simulink model "flightController"  (R2021b)
settings: Solver=ode3  StartTime=0  StopTime=10.0  FixedStep=Ts  RelTol=1e-3  EnableMultiTasking=on
settings Model: Creator=The MathWorks, Inc.  LastModifiedBy=Tiga
settings SolverCC: AlgebraicLoopSolver=TrustRegion  AutoInsertRateTranBlk=on
settings DataIOCC: SaveFormat=Array  ReturnWorkspaceOutputs=off
settings OptimizationCC: BlockReduction=off  DefaultParameterBehavior=Inlined  BufferReuse=off  LifeSpan=inf
settings DebuggingCC: AlgebraicLoopMsg=none  UnderspecifiedInitializationDetection=Classic  MergeDetectMultiDrivingBlocksExec=none  UnconnectedInputMsg=none  UnconnectedOutputMsg=none  UnconnectedLineMsg=none  AllowSymbolicDim=off  SymbolicDimsDataTypeCodeGenerationDiagnostic=none  SFUnexpectedBacktrackingDiag=warning  SFNoUnconditionalDefaultTransitionDiag=warning  SFExecutionAtInitializationDiag=none  SFMachineParentedDataDiag=warning  ArithmeticOperatorsInVariantConditions=warning
settings HardwareCC: ProdBitPerPointer=32  ProdBitPerSizeT=32  ProdBitPerPtrDiffT=32  ProdLargestAtomicFloat=None  ProdIntDivRoundTo=Undefined  ProdEndianess=Unspecified  ProdWordSize=32  ProdHWDeviceType=32-bit Generic
settings ModelReferenceCC: PropagateSignalLabelsOutOfModel=off
settings SFSimCC: SimUseLocalCustomCode=off
settings RTWCC: RTWUseLocalCustomCode=off
settings CodeAppCC: StateflowObjectComments=on
settings GRTTargetCC: TargetLangStandard=C89/C90 (ANSI)
settings ConfigComp: CovMetricSettings=dw  CovSaveCumulativeToWorkspaceVar=on  CovSaveSingleToWorkspaceVar=on  CovExternalEMLEnable=off

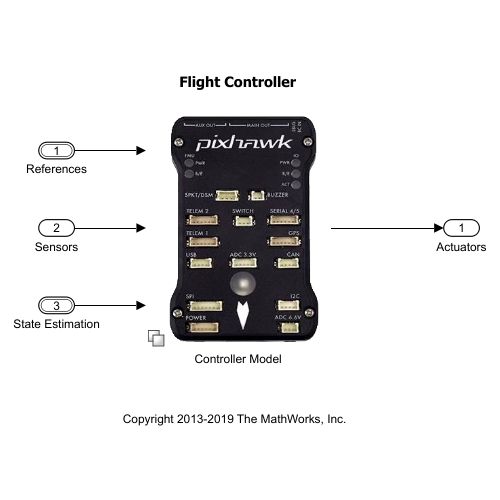
[thumbnail: Simulink's stored preview of the top-level diagram]
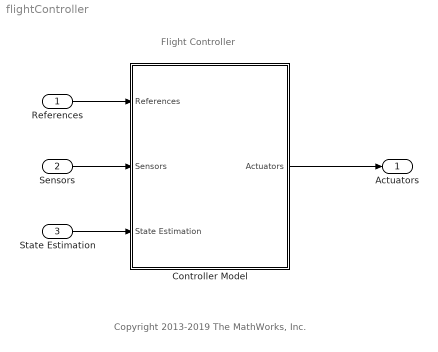
== system flightController ==
  note: Copyright 2013-2019 The MathWorks, Inc.
  note: Flight Controller
  References : Inport  OutDataTypeStr=Bus: ReferencesBus
  Sensors : Inport  Port=2
  State Estimation : Inport  Port=3  OutDataTypeStr=Bus: SensorsBus  BusOutputAsStruct=on
  Controller Model : Subsystem  Variant=on
      mask Display: image('pixhawk.png'); % Use "Edit Image" on toolstrip to change.
  Actuators : Outport  VectorParamsAs1DForOutWhenUnconnected=off
  wires:
  References/1 -> Controller Model/1(References)
  State Estimation/1 -> Controller Model/3(State Estimation)
  Controller Model/1(Actuators) -> Actuators/1
  Sensors/1 -> Controller Model/2(Sensors)

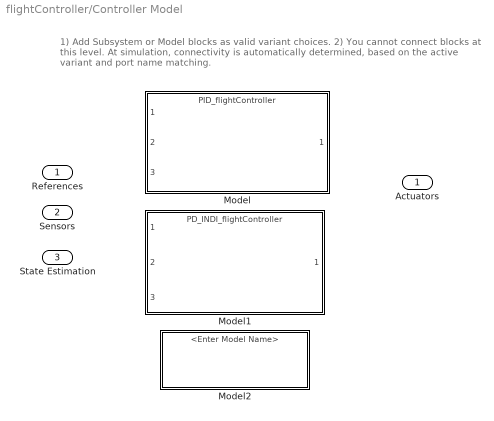
== system flightController/Controller Model ==
  note: 1) Add Subsystem or Model blocks as valid variant choices.
      | 2) You cannot connect blocks at this level. At simulation, connectivity is automatically
      | determined, based on the active variant and port name matching.
  References : Inport  OutDataTypeStr=Bus: ReferencesBus
  Sensors : Inport  Port=2
  State Estimation : Inport  Port=3  OutDataTypeStr=Bus: StatesBus
  Model : ModelReference  DisableCoverage=on  ModelNameDialog=PID_flightController.slx  VariantControl=true  ModelReferenceVersion=1.13
  Model1 : ModelReference  ModelNameDialog=PD_INDI_flightController.slx  VariantControl=false  ModelReferenceVersion=1.1
  Model2 : ModelReference  VariantControl=false
  Actuators : Outport
